simulink model "sampleModel1462"  (R2023a)
settings: Solver=VariableStepAuto  StartTime=0.0  StopTime=10.0  RelTol=1e-3
libraries: hdlsllib x2, simulink x1
settings Model: Creator=user1  LastModifiedBy=user1

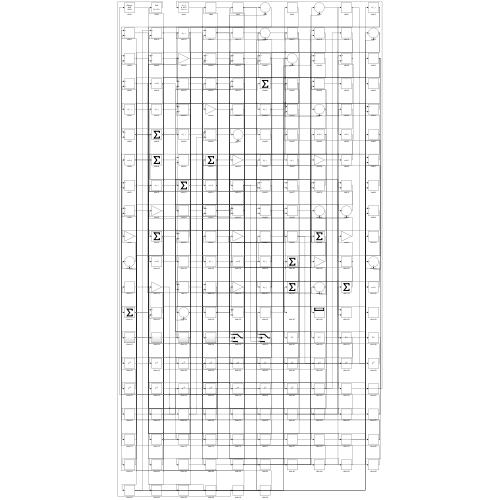
[thumbnail: Simulink's stored preview of the top-level diagram]
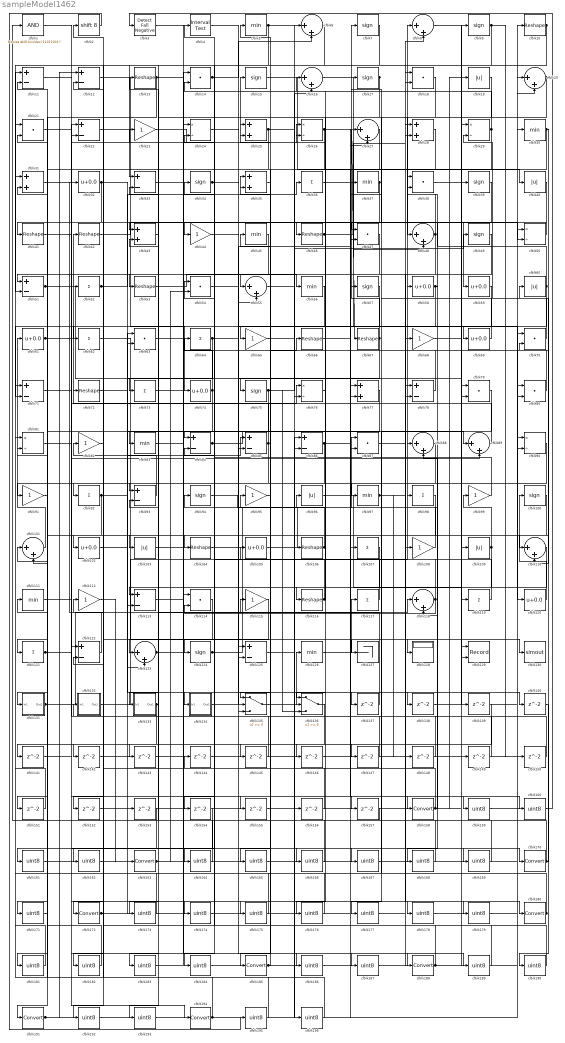
== system sampleModel1462 ==
  cfblk1 : simulink/Logic and Bit Operations/Bitwise Operator  logicop=AND  UseBitMask=on  BitMask=bin2dec('11011001')  BitMaskRealWorld=Stored Integer
      settings: LibrarySourceBlock=|
      | hdlsllib/Logic and Bit
      | Operations/Bitwise
      | Operator
  cfblk{10,13,41..42,46,53,66..67,72,104,106,116} (12 alike) : Reshape
  cfblk{7,9,15,17,34,39,49,57,75,94,100,124} (12 alike) : Signum
  cfblk{6,8,16,20,27,48,55,88..89,101,110,118,123} (13 alike) : Sum  Inputs=|++
  cfblk{32,58..59,61,69,74,102,105,120} (9 alike) : Bias  Bias=0.0  SaturateOnIntegerOverflow=off
  cfblk{19,40,60,96,103,109} (6 alike) : Abs  SaturateOnIntegerOverflow=off
  cfblk{36,52,62,64,73,92,98,107,117,119,121} (11 alike) : Sum  Inputs=+
  cfblk{23,44,65,68,82,91,95,99,108,112,115} (11 alike) : Gain
  cfblk{11..12,22,33,51,71,78,84..86,93,113,122,125} (14 alike) : Sum  Inputs=+-
  cfblk{5,30,37,45,56,83,97,111,126} (9 alike) : MinMax
  cfblk{14,18,21,38,47,54,63,70,79..80,87,114} (12 alike) : DotProduct  OutDataTypeStr=Inherit: Inherit via internal rule
  cfblk127 : Terminator
  cfblk128 : Display
  cfblk129 : Record  FileSettingsInternal="{\"entries\":[{\"content\":{\"excelSettings\":{\"content\":{},\"type\":\"Streamout.ExcelSettings\"}},\"type\":\"Streamout.FileSettingStorage\",\"uuid\":\"\"}],\"packageUris\":[\"http:\\/\\/schema.mathworks.com\\/mf0\\/streamout_blocks\\/R2020a\"],\"version\":\"1.0\"}"  Layout=[1 1]  SignalsInternal="{\"entries\":[{\"content\":{\"signals\":[{\"content\":{\"blockPath\":[],\"dimensions\":[1],\"domain\":\"\",\"lineColor\":\"#a2142f\",\"plots\":[1],\"port\":1,\"signalID\":855,\"signalName\":\"XY Graph:1\"},\"type\":\"RecordBlkView.Signal\",\"uuid\":\"\"},{\"content\":{\"blockPath\":[],\"dimensions\":[1],\"domain\":\"\",\"lineColor\":\"#139fff\",\"plots\":[1],\"port\":2,\"signalID\":858,\"signalName\":\"XY Graph:2\"},\"type\":\"RecordBlkView.Signal\",\"uuid\":\"\"}]},\"type\":\"RecordBlkView.InputSignals\",\"uuid\":\"\"}],\"packageUris\":[\"http:\\/\\/schema.mathworks.com\\/mf0\\/streamout_blocks\\/R2020a\"],\"version\":\"1.0\"}"  VisualizationBindings="{\"xyplotplugin\":{\"info\":[{\"series\":[{\"bindingParametersList\":[{\"parameter\":\"X-Axis\",\"signalID\":855,\"signalName\":\"XY Graph:1\"},{\"parameter\":\"Y-Axis\",\"signalID\":858,\"signalName\":\"XY Graph:2\"}],\"seriesID\":9135}],\"subplotID\":1}]}}"  CompatibilityTag=XY  st=-1
  cfblk130 : ToWorkspace  VariableName=simout  SaveFormat=Timeseries  SampleTime=-1
  cfblk131 : Subsystem
      settings: LibrarySourceBlock=|
      | hdlsllib/Ports &
      | Subsystems/Subsystem
  cfblk132 : Subsystem
      settings: LibrarySourceBlock=|
      | hdlsllib/Ports &
      | Subsystems/Subsystem
  cfblk133 : Subsystem
      settings: LibrarySourceBlock=|
      | hdlsllib/Ports &
      | Subsystems/Subsystem
  cfblk134 : Subsystem
      settings: LibrarySourceBlock=|
      | hdlsllib/Ports &
      | Subsystems/Subsystem
  cfblk135 : Switch  SaturateOnIntegerOverflow=off  InputSameDT=off
  cfblk136 : Switch  SaturateOnIntegerOverflow=off  InputSameDT=off
  cfblk{137..157} (21 alike) : Delay  SampleTime=1
  cfblk{158,163,170,172,180,185,188,191,194} (9 alike) : DataTypeConversion  SaturateOnIntegerOverflow=off  RndMeth=Floor
  cfblk{159..162,164..169,171,173..179,181..184,186..187,189..190,192..193,195..196} (30 alike) : DataTypeConversion  OutDataTypeStr=uint8  SaturateOnIntegerOverflow=off  RndMeth=Floor
  cfblk2 : ArithShift  BitShiftNumber=8
  cfblk{24,26,29,50,76,81,90} (7 alike) : Product  Inputs=*/  RndMeth=Zero  SaturateOnIntegerOverflow=on
  cfblk{25,28,31,35,43,77} (6 alike) : Sum
  cfblk3 : hdlsllib/Logic and Bit Operations/Detect Fall Negative  vinit=0  OutDataTypeStr=boolean
  cfblk4 : hdlsllib/Logic and Bit Operations/Interval Test  IntervalClosedRight=on  uplimit=0.5  IntervalClosedLeft=on  lowlimit=-0.5  OutDataTypeStr=boolean
  wires:
  cfblk85/1 -> cfblk42/1, cfblk101/2
  cfblk133/1(Out1) -> cfblk33/2, cfblk161/1
  cfblk53/1 -> cfblk56/1
  cfblk23/1 -> cfblk15/1
  cfblk122/1 -> cfblk32/1
  cfblk24/1 -> cfblk188/1
  cfblk22/1 -> cfblk74/1
  cfblk62/1 -> cfblk130/1
  cfblk94/1 -> cfblk96/1
  cfblk123/1 -> cfblk143/1, cfblk175/1
  cfblk38/1 -> cfblk39/1
  cfblk108/1 -> cfblk8/1
  cfblk68/1 -> cfblk129/1
  cfblk101/1 -> cfblk61/1
  cfblk124/1 -> cfblk87/1, cfblk47/2
  cfblk28/1 -> cfblk185/1
  cfblk12/1 -> cfblk46/1
  cfblk17/1 -> cfblk103/1, cfblk135/3
  cfblk10/1 -> cfblk102/1, cfblk22/2
  cfblk111/1 -> cfblk170/1
  cfblk126/1 -> cfblk117/1
  cfblk109/1 -> cfblk99/1, cfblk176/1
  cfblk74/1 -> cfblk83/1, cfblk64/1
  cfblk26/1 -> cfblk67/1, cfblk76/2
  cfblk75/1 -> cfblk136/3, cfblk16/2, cfblk154/1, cfblk173/1
  cfblk18/1 -> cfblk48/1
  cfblk3/1 -> cfblk158/1
  cfblk135/1 -> cfblk126/1
  cfblk40/1 -> cfblk59/1
  cfblk49/1 -> cfblk135/1
  cfblk67/1 -> cfblk7/1, cfblk85/2, cfblk145/1
  cfblk132/1(Out1) -> cfblk58/1
  cfblk16/1 -> cfblk120/1
  cfblk9/1 -> cfblk33/1, cfblk150/1
  cfblk55/1 -> cfblk49/1
  cfblk36/1 -> cfblk48/2
  cfblk27/1 -> cfblk191/1
  cfblk42/1 -> cfblk44/1
  cfblk86/1 -> cfblk113/1, cfblk159/1
  cfblk104/1 -> cfblk88/1
  cfblk58/1 -> cfblk86/2, cfblk118/2
  cfblk48/1 -> cfblk38/1, cfblk78/2
  cfblk105/1 -> cfblk57/1
  cfblk81/1 -> cfblk194/1
  cfblk84/1 -> cfblk89/1, cfblk55/2
  cfblk96/1 -> cfblk129/2
  cfblk120/1 -> cfblk100/1
  cfblk66/1 -> cfblk128/1
  cfblk131/1(Out1) -> cfblk118/1, cfblk101/1, cfblk76/1
  cfblk34/1 -> cfblk169/1, cfblk184/1
  cfblk15/1 -> cfblk40/1
  cfblk6/1 -> cfblk104/1
  cfblk46/1 -> cfblk8/2, cfblk136/1
  cfblk45/1 -> cfblk55/1
  cfblk98/1 -> cfblk121/1
  cfblk61/1 -> cfblk108/1, cfblk89/2
  cfblk117/1 -> cfblk5/1
  cfblk82/1 -> cfblk172/1
  cfblk25/1 -> cfblk92/1, cfblk50/2
  cfblk30/1 -> cfblk43/1, cfblk77/2, cfblk110/1, cfblk110/2
  cfblk64/1 -> cfblk4/1, cfblk113/2, cfblk187/1
  cfblk115/1 -> cfblk124/1
  cfblk103/1 -> cfblk35/1
  cfblk119/1 -> cfblk45/1
  cfblk13/1 -> cfblk73/1, cfblk51/1, cfblk186/1
  cfblk60/1 -> cfblk93/1, cfblk38/2
  cfblk31/1 -> cfblk180/1
  cfblk35/1 -> cfblk75/1
  cfblk50/1 -> cfblk41/1
  cfblk7/1 -> cfblk123/1
  cfblk118/1 -> cfblk114/2, cfblk105/1
  cfblk56/1 -> cfblk71/2
  cfblk113/1 -> cfblk66/1
  cfblk37/1 -> cfblk84/1, cfblk182/1
  cfblk116/1 -> cfblk26/1, cfblk84/2
  cfblk78/1 -> cfblk16/1
  cfblk93/1 -> cfblk2/1
  cfblk72/1 -> cfblk87/2
  cfblk69/1 -> cfblk37/1
  cfblk106/1 -> cfblk25/1, cfblk94/1
  cfblk79/1 -> cfblk97/1
  cfblk59/1 -> cfblk65/1
  cfblk32/1 -> cfblk91/1, cfblk134/1(In1)
  cfblk14/1 -> cfblk69/1, cfblk6/2
  cfblk121/1 -> cfblk23/1, cfblk155/1
  cfblk77/1 -> cfblk131/1(In1)
  cfblk57/1 -> cfblk135/2
  cfblk51/1 -> cfblk109/1, cfblk12/1
  cfblk99/1 -> cfblk34/1
  cfblk41/1 -> cfblk26/2
  cfblk134/1(Out1) -> cfblk125/1
  cfblk4/1 -> cfblk79/2
  cfblk102/1 -> cfblk85/1
  cfblk92/1 -> cfblk136/2, cfblk141/1
  cfblk29/1 -> cfblk62/1, cfblk14/2
  cfblk70/1 -> cfblk29/2
  cfblk97/1 -> cfblk148/1, cfblk179/1
  cfblk5/1 -> cfblk6/1, cfblk51/2, cfblk138/1
  cfblk44/1 -> cfblk125/2
  cfblk1/1 -> cfblk122/1
  cfblk89/1 -> cfblk54/1
  cfblk112/1 -> cfblk163/1
  cfblk20/1 -> cfblk53/1, cfblk47/1
  cfblk19/1 -> cfblk116/1
  cfblk43/1 -> cfblk133/1(In1)
  cfblk80/1 -> cfblk25/2
  cfblk125/1 -> cfblk127/1
  cfblk52/1 -> cfblk123/2, cfblk36/1
  cfblk87/1 -> cfblk68/1
  cfblk54/1 -> cfblk137/1
  cfblk137/1 -> cfblk93/2
  cfblk138/1 -> cfblk20/1
  cfblk8/1 -> cfblk139/1
  cfblk83/1 -> cfblk140/1
  cfblk136/1 -> cfblk142/1
  cfblk142/1 -> cfblk79/1
  cfblk143/1 -> cfblk80/2
  cfblk144/1 -> cfblk18/1
  cfblk145/1 -> cfblk122/2
  cfblk76/1 -> cfblk146/1
  cfblk146/1 -> cfblk70/1
  cfblk100/1 -> cfblk147/1
  cfblk147/1 -> cfblk22/1
  cfblk148/1 -> cfblk14/1
  cfblk149/1 -> cfblk43/2
  cfblk150/1 -> cfblk88/2
  cfblk47/1 -> cfblk151/1
  cfblk151/1 -> cfblk71/1
  cfblk114/1 -> cfblk152/1
  cfblk152/1 -> cfblk29/1
  cfblk65/1 -> cfblk156/1
  cfblk156/1 -> cfblk86/1
  cfblk73/1 -> cfblk157/1
  cfblk157/1 -> cfblk1/1
  cfblk158/1 -> cfblk98/1, cfblk12/2, cfblk19/1
  cfblk159/1 -> cfblk3/1
  cfblk63/1 -> cfblk160/1
  cfblk160/1 -> cfblk70/2
  cfblk161/1 -> cfblk63/1
  cfblk153/1 -> cfblk162/1
  cfblk162/1 -> cfblk63/2
  cfblk163/1 -> cfblk119/1, cfblk54/2
  cfblk110/1 -> cfblk164/1
  cfblk164/1 -> cfblk112/1
  cfblk95/1 -> cfblk165/1
  cfblk165/1 -> cfblk149/1
  cfblk33/1 -> cfblk166/1
  cfblk166/1 -> cfblk95/1
  cfblk21/1 -> cfblk167/1
  cfblk167/1 -> cfblk80/1
  cfblk39/1 -> cfblk168/1
  cfblk168/1 -> cfblk21/1
  cfblk169/1 -> cfblk21/2
  cfblk170/1 -> cfblk13/1, cfblk60/1
  cfblk91/1 -> cfblk171/1
  cfblk171/1 -> cfblk111/1
  cfblk172/1 -> cfblk153/1, cfblk77/1
  cfblk173/1 -> cfblk82/1
  cfblk11/1 -> cfblk174/1
  cfblk174/1 -> cfblk144/1
  cfblk175/1 -> cfblk11/1
  cfblk176/1 -> cfblk11/2
  cfblk90/1 -> cfblk177/1
  cfblk177/1 -> cfblk18/2
  cfblk141/1 -> cfblk178/1
  cfblk178/1 -> cfblk90/1
  cfblk179/1 -> cfblk90/2
  cfblk180/1 -> cfblk17/1, cfblk35/2
  cfblk154/1 -> cfblk181/1
  cfblk181/1 -> cfblk31/1
  cfblk182/1 -> cfblk31/2
  cfblk107/1 -> cfblk183/1
  cfblk183/1 -> cfblk114/1
  cfblk184/1 -> cfblk107/1
  cfblk185/1 -> cfblk115/1, cfblk78/1, cfblk9/1
  cfblk186/1 -> cfblk28/1
  cfblk187/1 -> cfblk28/2
  cfblk188/1 -> cfblk132/1(In1), cfblk30/1
  cfblk71/1 -> cfblk189/1
  cfblk189/1 -> cfblk24/1
  cfblk140/1 -> cfblk190/1
  cfblk190/1 -> cfblk24/2
  cfblk191/1 -> cfblk50/1, cfblk106/1, cfblk52/1, cfblk10/1
  cfblk88/1 -> cfblk192/1
  cfblk192/1 -> cfblk27/1
  cfblk139/1 -> cfblk193/1
  cfblk193/1 -> cfblk27/2
  cfblk194/1 -> cfblk20/2, cfblk72/1
  cfblk2/1 -> cfblk195/1
  cfblk195/1 -> cfblk81/1
  cfblk155/1 -> cfblk196/1
  cfblk196/1 -> cfblk81/2

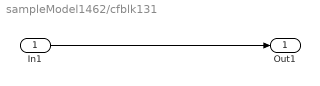
== system sampleModel1462/cfblk131 ==
  In1 : Inport
  Out1 : Outport
  wires:
  In1/1 -> Out1/1

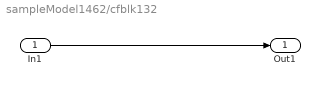
== system sampleModel1462/cfblk132 ==
  In1 : Inport
  Out1 : Outport
  wires:
  In1/1 -> Out1/1

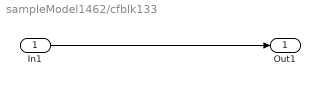
== system sampleModel1462/cfblk133 ==
  In1 : Inport
  Out1 : Outport
  wires:
  In1/1 -> Out1/1

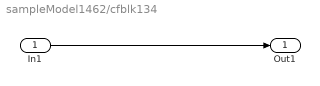
== system sampleModel1462/cfblk134 ==
  In1 : Inport
  Out1 : Outport
  wires:
  In1/1 -> Out1/1
